simulink model "experiment_simulation"  (R2023b)
settings: Solver=VariableStepAuto  StartTime=0.0  StopTime=27  RelTol=1e-3
InitFcn:
  | parameters
model workspace (MAT data in the model file):
  trajectory_a = [-1.52409846931 0.800900294758 0.522291166812 0.881049446282 0.615681685123 0.846225707965 -1.91228070877 1.70613035573 -0.416782684687 1.94182780206 0.715113366686 0.630917086666 ... (70 elements, 7x10)]
  trajectory_b = [1.63785922603 1.06519745333 0.917286904974 -0.0990593700309 -1.33458996905 1.44935684592 -1.71486047215 -1.76858838765 1.00521664875 1.43938283234 1.2212819449 -1.40157163353 ... (70 elements, 7x10)]
values from neighbouring files (symbols this model uses):
  m = length(U)-1    [bspline_findspan.m]
  param_robot = load_mu(param_robot, mu)    [parameters.m]
undefined symbols (not defined in the file or in its folder): par, param_initial_condition, param_sensor, X, Y, Z
libraries: nesl_utility x308, sm_lib x269, simulink_extras x1
(part 3 of 4)

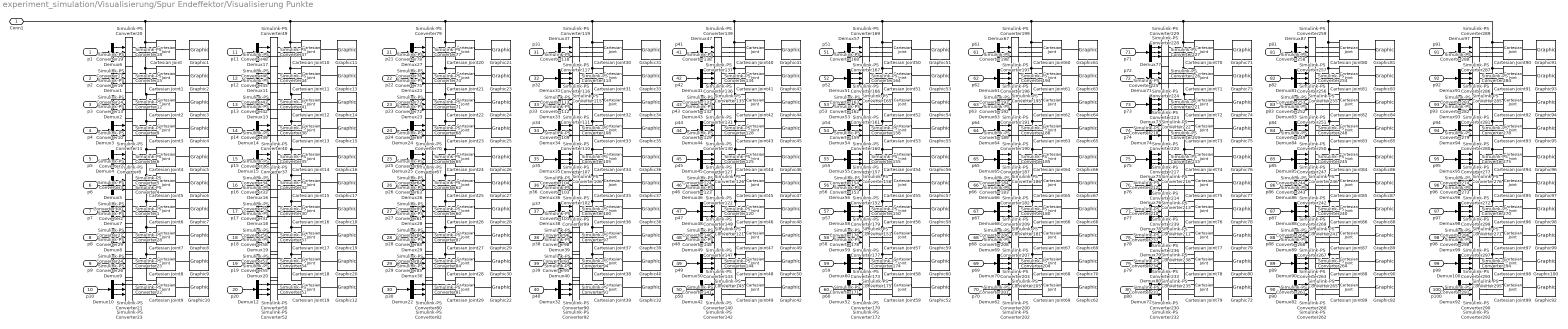
== system experiment_simulation/Visualisierung/Spur Endeffektor/Visualisierung Punkte ==
  p1 : Inport
  p2 : Inport  Port=2
  p3 : Inport  Port=3
  p4 : Inport  Port=4
  p5 : Inport  Port=5
  p6 : Inport  Port=6
  p7 : Inport  Port=7
  p8 : Inport  Port=8
  p9 : Inport  Port=9
  p10 : Inport  Port=10
  p11 : Inport  Port=11
  p12 : Inport  Port=12
  p13 : Inport  Port=13
  p14 : Inport  Port=14
  p15 : Inport  Port=15
  p16 : Inport  Port=16
  p17 : Inport  Port=17
  p18 : Inport  Port=18
  p19 : Inport  Port=19
  p20 : Inport  Port=20
  p21 : Inport  Port=21
  p22 : Inport  Port=22
  p23 : Inport  Port=23
  p24 : Inport  Port=24
  p25 : Inport  Port=25
  p26 : Inport  Port=26
  p27 : Inport  Port=27
  p28 : Inport  Port=28
  p29 : Inport  Port=29
  p30 : Inport  Port=30
  p31 : Inport  Port=31
  p32 : Inport  Port=32
  p33 : Inport  Port=33
  p34 : Inport  Port=34
  p35 : Inport  Port=35
  p36 : Inport  Port=36
  p37 : Inport  Port=37
  p38 : Inport  Port=38
  p39 : Inport  Port=39
  p40 : Inport  Port=40
  p41 : Inport  Port=41
  p42 : Inport  Port=42
  p43 : Inport  Port=43
  p44 : Inport  Port=44
  p45 : Inport  Port=45
  p46 : Inport  Port=46
  p47 : Inport  Port=47
  p48 : Inport  Port=48
  p49 : Inport  Port=49
  p50 : Inport  Port=50
  p51 : Inport  Port=51
  p52 : Inport  Port=52
  p53 : Inport  Port=53
  p54 : Inport  Port=54
  p55 : Inport  Port=55
  p56 : Inport  Port=56
  p57 : Inport  Port=57
  p58 : Inport  Port=58
  p59 : Inport  Port=59
  p60 : Inport  Port=60
  p61 : Inport  Port=61
  p62 : Inport  Port=62
  p63 : Inport  Port=63
  p64 : Inport  Port=64
  p65 : Inport  Port=65
  p66 : Inport  Port=66
  p67 : Inport  Port=67
  p68 : Inport  Port=68
  p69 : Inport  Port=69
  p70 : Inport  Port=70
  p71 : Inport  Port=71
  p72 : Inport  Port=72
  p73 : Inport  Port=73
  p74 : Inport  Port=74
  p75 : Inport  Port=75
  p76 : Inport  Port=76
  p77 : Inport  Port=77
  p78 : Inport  Port=78
  p79 : Inport  Port=79
  p80 : Inport  Port=80
  p81 : Inport  Port=81
  p82 : Inport  Port=82
  p83 : Inport  Port=83
  p84 : Inport  Port=84
  p85 : Inport  Port=85
  p86 : Inport  Port=86
  p87 : Inport  Port=87
  p88 : Inport  Port=88
  p89 : Inport  Port=89
  p90 : Inport  Port=90
  p91 : Inport  Port=91
  p92 : Inport  Port=92
  p93 : Inport  Port=93
  p94 : Inport  Port=94
  p95 : Inport  Port=95
  p96 : Inport  Port=96
  p97 : Inport  Port=97
  p98 : Inport  Port=98
  p99 : Inport  Port=99
  p100 : Inport  Port=100
  Cartesian Joint{,1..99} (100 alike) : sm_lib/Joints/Cartesian Joint  JointMode=Normal  SenseConstraintForce=off  SenseConstraintForceX=off  SenseConstraintForceY=off  SenseConstraintForceZ=off  SenseConstraintTorque=off  SenseConstraintTorqueX=off  SenseConstraintTorqueY=off  SenseConstraintTorqueZ=off  SenseTotalForce=off  SenseTotalForceX=off  SenseTotalForceY=off  SenseTotalForceZ=off  SenseTotalTorque=off  SenseTotalTorqueX=off  SenseTotalTorqueY=off  SenseTotalTorqueZ=off  CompositeWrenchDir=FollowerOnBase  CompositeWrenchFrame=BaseFrame  PxEquilibriumPosition=0  PxEquilibriumPositionUnits=m  PxSpringStiffness=0  PxSpringStiffnessUnits=N/m  PxDampingCoefficient=0  PxDampingCoefficientUnits=N/(m/s)  PxTorqueActuationMode=ComputedTorque  PxMotionActuationMode=InputMotion  PxSensePosition=off  PxSenseVelocity=off  PxSenseAcceleration=off  PxSenseTorqueForce=off  PxSenseLowerLimitTorqueForce=off  PxSenseUpperLimitTorqueForce=off  PxLowerLimitSpecify=off  PxLowerLimitBound=-1  PxLowerLimitBoundUnits=m  PxLowerLimitStiffness=1e6  PxLowerLimitStiffnessUnits=N/m  PxLowerLimitDamping=1e3  PxLowerLimitDampingUnits=N/(m/s)  PxLowerLimitTransitionRegionWidth=1e-4  PxLowerLimitTransitionRegionWidthUnits=m  PxUpperLimitSpecify=off  PxUpperLimitBound=1  PxUpperLimitBoundUnits=m  PxUpperLimitStiffness=1e6  PxUpperLimitStiffnessUnits=N/m  PxUpperLimitDamping=1e3  PxUpperLimitDampingUnits=N/(m/s)  PxUpperLimitTransitionRegionWidth=1e-4  PxUpperLimitTransitionRegionWidthUnits=m  PxPositionTargetSpecify=off  PxPositionTargetPriority=High  PxPositionTargetValue=0  PxPositionTargetValueUnits=m  PxVelocityTargetSpecify=off  PxVelocityTargetPriority=High  PxVelocityTargetValue=0  PxVelocityTargetValueUnits=m/s  PyEquilibriumPosition=0  PyEquilibriumPositionUnits=m  PySpringStiffness=0  PySpringStiffnessUnits=N/m  PyDampingCoefficient=0  PyDampingCoefficientUnits=N/(m/s)  PyTorqueActuationMode=ComputedTorque  PyMotionActuationMode=InputMotion  PySensePosition=off  PySenseVelocity=off  PySenseAcceleration=off  PySenseTorqueForce=off  PySenseLowerLimitTorqueForce=off  PySenseUpperLimitTorqueForce=off  PyLowerLimitSpecify=off  PyLowerLimitBound=-1  PyLowerLimitBoundUnits=m  PyLowerLimitStiffness=1e6  PyLowerLimitStiffnessUnits=N/m  PyLowerLimitDamping=1e3  PyLowerLimitDampingUnits=N/(m/s)  PyLowerLimitTransitionRegionWidth=1e-4  PyLowerLimitTransitionRegionWidthUnits=m  PyUpperLimitSpecify=off  PyUpperLimitBound=1  PyUpperLimitBoundUnits=m  PyUpperLimitStiffness=1e6  PyUpperLimitStiffnessUnits=N/m  PyUpperLimitDamping=1e3  PyUpperLimitDampingUnits=N/(m/s)  PyUpperLimitTransitionRegionWidth=1e-4  PyUpperLimitTransitionRegionWidthUnits=m  PyPositionTargetSpecify=off  PyPositionTargetPriority=High  PyPositionTargetValue=0  PyPositionTargetValueUnits=m  PyVelocityTargetSpecify=off  PyVelocityTargetPriority=High  PyVelocityTargetValue=0  PyVelocityTargetValueUnits=m/s  PzEquilibriumPosition=0  PzEquilibriumPositionUnits=m  PzSpringStiffness=0  PzSpringStiffnessUnits=N/m  PzDampingCoefficient=0  PzDampingCoefficientUnits=N/(m/s)  PzTorqueActuationMode=ComputedTorque  PzMotionActuationMode=InputMotion  PzSensePosition=off  PzSenseVelocity=off  PzSenseAcceleration=off  PzSenseTorqueForce=off  PzSenseLowerLimitTorqueForce=off  PzSenseUpperLimitTorqueForce=off  PzLowerLimitSpecify=off  PzLowerLimitBound=-1  PzLowerLimitBoundUnits=m  PzLowerLimitStiffness=1e6  PzLowerLimitStiffnessUnits=N/m  PzLowerLimitDamping=1e3  PzLowerLimitDampingUnits=N/(m/s)  PzLowerLimitTransitionRegionWidth=1e-4  PzLowerLimitTransitionRegionWidthUnits=m  PzUpperLimitSpecify=off  PzUpperLimitBound=1  PzUpperLimitBoundUnits=m  PzUpperLimitStiffness=1e6  PzUpperLimitStiffnessUnits=N/m  PzUpperLimitDamping=1e3  PzUpperLimitDampingUnits=N/(m/s)  PzUpperLimitTransitionRegionWidth=1e-4  PzUpperLimitTransitionRegionWidthUnits=m  PzPositionTargetSpecify=off  PzPositionTargetPriority=High  PzPositionTargetValue=0  PzPositionTargetValueUnits=m  PzVelocityTargetSpecify=off  PzVelocityTargetPriority=High  PzVelocityTargetValue=0  PzVelocityTargetValueUnits=m/s
  Demux{1..100} (100 alike) : Demux  Outputs=3
  Graphic{1..100} (100 alike) : sm_lib/Body Elements/Graphic  GraphicType=Marker  MarkerShape=Sphere  MarkerSize=par.vis_point.pix  GraphicVisPropType=SimpleVisualProperties  GraphicDiffuseColor=par.vis_point.col  GraphicSpecularColor=[0.5 0.5 0.5 1.0]  GraphicAmbientColor=[0.15 0.15 0.15 1.0]  GraphicEmissiveColor=[0.0 0.0 0.0 1.0]  GraphicShininess=75  GraphicOpacity=par.vis_point.opa
  Simulink-PS Converter{1..300} (300 alike) : nesl_utility/Simulink-PS Converter  PhysicalDomain=network_engine_domain  SubClassName=ps_input  LeftPortType=input  RightPortType=output  PseudoPeriodic=off  Frequencies=[]  NoiseDistribution=none  NoiseParameters=[]  Unit=1  AffineConversion=off  FilteringAndDerivatives=zero  SimscapeFilterOrder=2  InputFilterTimeConstant=0.001  UdotUserProvided=0
  Conn1 : PMIOPort  Side=Left
  wires:
  Demux6/2 -> Simulink-PS Converter18/1
  Demux6/3 -> Simulink-PS Converter19/1
  Demux6/1 -> Simulink-PS Converter20/1
  p1/1 -> Demux6/1
  Demux1/3 -> Simulink-PS Converter16/1
  Demux1/1 -> Simulink-PS Converter17/1
  Demux1/2 -> Simulink-PS Converter15/1
  p2/1 -> Demux1/1
  Demux2/3 -> Simulink-PS Converter13/1
  Demux2/1 -> Simulink-PS Converter14/1
  Demux2/2 -> Simulink-PS Converter12/1
  p3/1 -> Demux2/1
  Demux3/3 -> Simulink-PS Converter10/1
  Demux3/1 -> Simulink-PS Converter11/1
  Demux3/2 -> Simulink-PS Converter9/1
  p4/1 -> Demux3/1
  Demux4/3 -> Simulink-PS Converter7/1
  Demux4/1 -> Simulink-PS Converter8/1
  Demux4/2 -> Simulink-PS Converter6/1
  p5/1 -> Demux4/1
  Demux5/3 -> Simulink-PS Converter4/1
  Demux5/1 -> Simulink-PS Converter5/1
  Demux5/2 -> Simulink-PS Converter3/1
  p6/1 -> Demux5/1
  Demux7/3 -> Simulink-PS Converter2/1
  Demux7/1 -> Simulink-PS Converter300/1
  Demux7/2 -> Simulink-PS Converter1/1
  p7/1 -> Demux7/1
  Demux8/3 -> Simulink-PS Converter29/1
  Demux8/1 -> Simulink-PS Converter27/1
  Demux8/2 -> Simulink-PS Converter28/1
  p8/1 -> Demux8/1
  Demux9/3 -> Simulink-PS Converter26/1
  Demux9/1 -> Simulink-PS Converter24/1
  Demux9/2 -> Simulink-PS Converter25/1
  p9/1 -> Demux9/1
  Demux10/3 -> Simulink-PS Converter23/1
  Demux10/1 -> Simulink-PS Converter21/1
  Demux10/2 -> Simulink-PS Converter22/1
  p10/1 -> Demux10/1
  Demux16/2 -> Simulink-PS Converter32/1
  Demux16/1 -> Simulink-PS Converter34/1
  p16/1 -> Demux16/1
  p20/1 -> Demux12/1
  Demux12/2 -> Simulink-PS Converter51/1
  Demux12/1 -> Simulink-PS Converter50/1
  Demux12/3 -> Simulink-PS Converter52/1
  Demux17/1 -> Simulink-PS Converter49/1
  Demux17/3 -> Simulink-PS Converter48/1
  Demux17/2 -> Simulink-PS Converter47/1
  p11/1 -> Demux17/1
  Demux19/3 -> Simulink-PS Converter58/1
  p18/1 -> Demux19/1
  Demux11/2 -> Simulink-PS Converter44/1
  Demux11/1 -> Simulink-PS Converter46/1
  Demux19/2 -> Simulink-PS Converter57/1
  Demux11/3 -> Simulink-PS Converter45/1
  Demux19/1 -> Simulink-PS Converter56/1
  Demux15/1 -> Simulink-PS Converter37/1
  p12/1 -> Demux11/1
  p15/1 -> Demux15/1
  p17/1 -> Demux18/1
  Demux18/2 -> Simulink-PS Converter30/1
  Demux18/3 -> Simulink-PS Converter31/1
  Demux18/1 -> Simulink-PS Converter59/1
  Demux13/2 -> Simulink-PS Converter41/1
  Demux15/2 -> Simulink-PS Converter35/1
  Demux14/3 -> Simulink-PS Converter39/1
  Demux13/1 -> Simulink-PS Converter43/1
  Demux13/3 -> Simulink-PS Converter42/1
  Demux14/2 -> Simulink-PS Converter38/1
  Demux16/3 -> Simulink-PS Converter33/1
  p13/1 -> Demux13/1
  p19/1 -> Demux20/1
  Demux20/3 -> Simulink-PS Converter55/1
  p14/1 -> Demux14/1
  Demux20/1 -> Simulink-PS Converter53/1
  Demux14/1 -> Simulink-PS Converter40/1
  Demux20/2 -> Simulink-PS Converter54/1
  Demux15/3 -> Simulink-PS Converter36/1
  Demux26/2 -> Simulink-PS Converter62/1
  Demux26/1 -> Simulink-PS Converter64/1
  p26/1 -> Demux26/1
  p30/1 -> Demux22/1
  Demux22/2 -> Simulink-PS Converter81/1
  Demux22/1 -> Simulink-PS Converter80/1
  Demux22/3 -> Simulink-PS Converter82/1
  Demux27/1 -> Simulink-PS Converter79/1
  Demux27/3 -> Simulink-PS Converter78/1
  Demux27/2 -> Simulink-PS Converter77/1
  p21/1 -> Demux27/1
  Demux29/3 -> Simulink-PS Converter88/1
  p28/1 -> Demux29/1
  Demux21/2 -> Simulink-PS Converter74/1
  Demux21/1 -> Simulink-PS Converter76/1
  Demux29/2 -> Simulink-PS Converter87/1
  Demux21/3 -> Simulink-PS Converter75/1
  Demux29/1 -> Simulink-PS Converter86/1
  Demux25/1 -> Simulink-PS Converter67/1
  p22/1 -> Demux21/1
  p25/1 -> Demux25/1
  p27/1 -> Demux28/1
  Demux28/2 -> Simulink-PS Converter60/1
  Demux28/3 -> Simulink-PS Converter61/1
  Demux28/1 -> Simulink-PS Converter89/1
  Demux23/2 -> Simulink-PS Converter71/1
  Demux25/2 -> Simulink-PS Converter65/1
  Demux24/3 -> Simulink-PS Converter69/1
  Demux23/1 -> Simulink-PS Converter73/1
  Demux23/3 -> Simulink-PS Converter72/1
  Demux24/2 -> Simulink-PS Converter68/1
  Demux26/3 -> Simulink-PS Converter63/1
  p23/1 -> Demux23/1
  p29/1 -> Demux30/1
  Demux30/3 -> Simulink-PS Converter85/1
  p24/1 -> Demux24/1
  Demux30/1 -> Simulink-PS Converter83/1
  Demux24/1 -> Simulink-PS Converter70/1
  Demux30/2 -> Simulink-PS Converter84/1
  Demux25/3 -> Simulink-PS Converter66/1
  Demux36/2 -> Simulink-PS Converter102/1
  Demux36/1 -> Simulink-PS Converter104/1
  p36/1 -> Demux36/1
  p40/1 -> Demux32/1
  Demux32/2 -> Simulink-PS Converter91/1
  Demux32/1 -> Simulink-PS Converter90/1
  Demux32/3 -> Simulink-PS Converter92/1
  Demux37/1 -> Simulink-PS Converter119/1
  Demux37/3 -> Simulink-PS Converter118/1
  Demux37/2 -> Simulink-PS Converter117/1
  p31/1 -> Demux37/1
  Demux39/3 -> Simulink-PS Converter98/1
  p38/1 -> Demux39/1
  Demux31/2 -> Simulink-PS Converter114/1
  Demux31/1 -> Simulink-PS Converter116/1
  Demux39/2 -> Simulink-PS Converter97/1
  Demux31/3 -> Simulink-PS Converter115/1
  Demux39/1 -> Simulink-PS Converter96/1
  Demux35/1 -> Simulink-PS Converter107/1
  p32/1 -> Demux31/1
  p35/1 -> Demux35/1
  p37/1 -> Demux38/1
  Demux38/2 -> Simulink-PS Converter100/1
  Demux38/3 -> Simulink-PS Converter101/1
  Demux38/1 -> Simulink-PS Converter99/1
  Demux33/2 -> Simulink-PS Converter111/1
  Demux35/2 -> Simulink-PS Converter105/1
  Demux34/3 -> Simulink-PS Converter109/1
  Demux33/1 -> Simulink-PS Converter113/1
  Demux33/3 -> Simulink-PS Converter112/1
  Demux34/2 -> Simulink-PS Converter108/1
  Demux36/3 -> Simulink-PS Converter103/1
  p33/1 -> Demux33/1
  p39/1 -> Demux40/1
  Demux40/3 -> Simulink-PS Converter95/1
  p34/1 -> Demux34/1
  Demux40/1 -> Simulink-PS Converter93/1
  Demux34/1 -> Simulink-PS Converter110/1
  Demux40/2 -> Simulink-PS Converter94/1
  Demux35/3 -> Simulink-PS Converter106/1
  Demux46/2 -> Simulink-PS Converter122/1
  Demux46/1 -> Simulink-PS Converter124/1
  p46/1 -> Demux46/1
  p50/1 -> Demux42/1
  Demux42/2 -> Simulink-PS Converter141/1
  Demux42/1 -> Simulink-PS Converter140/1
  Demux42/3 -> Simulink-PS Converter142/1
  Demux47/1 -> Simulink-PS Converter139/1
  Demux47/3 -> Simulink-PS Converter138/1
  Demux47/2 -> Simulink-PS Converter137/1
  p41/1 -> Demux47/1
  Demux49/3 -> Simulink-PS Converter148/1
  p48/1 -> Demux49/1
  Demux41/2 -> Simulink-PS Converter134/1
  Demux41/1 -> Simulink-PS Converter136/1
  Demux49/2 -> Simulink-PS Converter147/1
  Demux41/3 -> Simulink-PS Converter135/1
  Demux49/1 -> Simulink-PS Converter146/1
  Demux45/1 -> Simulink-PS Converter127/1
  p42/1 -> Demux41/1
  p45/1 -> Demux45/1
  p47/1 -> Demux48/1
  Demux48/2 -> Simulink-PS Converter120/1
  Demux48/3 -> Simulink-PS Converter121/1
  Demux48/1 -> Simulink-PS Converter149/1
  Demux43/2 -> Simulink-PS Converter131/1
  Demux45/2 -> Simulink-PS Converter125/1
  Demux44/3 -> Simulink-PS Converter129/1
  Demux43/1 -> Simulink-PS Converter133/1
  Demux43/3 -> Simulink-PS Converter132/1
  Demux44/2 -> Simulink-PS Converter128/1
  Demux46/3 -> Simulink-PS Converter123/1
  p43/1 -> Demux43/1
  p49/1 -> Demux50/1
  Demux50/3 -> Simulink-PS Converter145/1
  p44/1 -> Demux44/1
  Demux50/1 -> Simulink-PS Converter143/1
  Demux44/1 -> Simulink-PS Converter130/1
  Demux50/2 -> Simulink-PS Converter144/1
  Demux45/3 -> Simulink-PS Converter126/1
  Demux56/2 -> Simulink-PS Converter152/1
  Demux56/1 -> Simulink-PS Converter154/1
  p56/1 -> Demux56/1
  p60/1 -> Demux52/1
  Demux52/2 -> Simulink-PS Converter171/1
  Demux52/1 -> Simulink-PS Converter170/1
  Demux52/3 -> Simulink-PS Converter172/1
  Demux57/1 -> Simulink-PS Converter169/1
  Demux57/3 -> Simulink-PS Converter168/1
  Demux57/2 -> Simulink-PS Converter167/1
  p51/1 -> Demux57/1
  Demux59/3 -> Simulink-PS Converter178/1
  p58/1 -> Demux59/1
  Demux51/2 -> Simulink-PS Converter164/1
  Demux51/1 -> Simulink-PS Converter166/1
  Demux59/2 -> Simulink-PS Converter177/1
  Demux51/3 -> Simulink-PS Converter165/1
  Demux59/1 -> Simulink-PS Converter176/1
  Demux55/1 -> Simulink-PS Converter157/1
  p52/1 -> Demux51/1
  p55/1 -> Demux55/1
  p57/1 -> Demux58/1
  Demux58/2 -> Simulink-PS Converter150/1
  Demux58/3 -> Simulink-PS Converter151/1
  Demux58/1 -> Simulink-PS Converter179/1
  Demux53/2 -> Simulink-PS Converter161/1
  Demux55/2 -> Simulink-PS Converter155/1
  Demux54/3 -> Simulink-PS Converter159/1
  Demux53/1 -> Simulink-PS Converter163/1
  Demux53/3 -> Simulink-PS Converter162/1
  Demux54/2 -> Simulink-PS Converter158/1
  Demux56/3 -> Simulink-PS Converter153/1
  p53/1 -> Demux53/1
  p59/1 -> Demux60/1
  Demux60/3 -> Simulink-PS Converter175/1
  p54/1 -> Demux54/1
  Demux60/1 -> Simulink-PS Converter173/1
  Demux54/1 -> Simulink-PS Converter160/1
  Demux60/2 -> Simulink-PS Converter174/1
  Demux55/3 -> Simulink-PS Converter156/1
  Demux66/2 -> Simulink-PS Converter182/1
  Demux66/1 -> Simulink-PS Converter184/1
  p66/1 -> Demux66/1
  p70/1 -> Demux62/1
  Demux62/2 -> Simulink-PS Converter201/1
  Demux62/1 -> Simulink-PS Converter200/1
  Demux62/3 -> Simulink-PS Converter202/1
  Demux67/1 -> Simulink-PS Converter199/1
  Demux67/3 -> Simulink-PS Converter198/1
  Demux67/2 -> Simulink-PS Converter197/1
  p61/1 -> Demux67/1
  Demux69/3 -> Simulink-PS Converter208/1
  p68/1 -> Demux69/1
  Demux61/2 -> Simulink-PS Converter194/1
  Demux61/1 -> Simulink-PS Converter196/1
  Demux69/2 -> Simulink-PS Converter207/1
  Demux61/3 -> Simulink-PS Converter195/1
  Demux69/1 -> Simulink-PS Converter206/1
  Demux65/1 -> Simulink-PS Converter187/1
  p62/1 -> Demux61/1
  p65/1 -> Demux65/1
  p67/1 -> Demux68/1
  Demux68/2 -> Simulink-PS Converter180/1
  Demux68/3 -> Simulink-PS Converter181/1
  Demux68/1 -> Simulink-PS Converter209/1
  Demux63/2 -> Simulink-PS Converter191/1
  Demux65/2 -> Simulink-PS Converter185/1
  Demux64/3 -> Simulink-PS Converter189/1
  Demux63/1 -> Simulink-PS Converter193/1
  Demux63/3 -> Simulink-PS Converter192/1
  Demux64/2 -> Simulink-PS Converter188/1
  Demux66/3 -> Simulink-PS Converter183/1
  p63/1 -> Demux63/1
  p69/1 -> Demux70/1
  Demux70/3 -> Simulink-PS Converter205/1
  p64/1 -> Demux64/1
  Demux70/1 -> Simulink-PS Converter203/1
  Demux64/1 -> Simulink-PS Converter190/1
  Demux70/2 -> Simulink-PS Converter204/1
  Demux65/3 -> Simulink-PS Converter186/1
  Demux76/2 -> Simulink-PS Converter212/1
  Demux76/1 -> Simulink-PS Converter214/1
  p76/1 -> Demux76/1
  p80/1 -> Demux72/1
  Demux72/2 -> Simulink-PS Converter231/1
  Demux72/1 -> Simulink-PS Converter230/1
  Demux72/3 -> Simulink-PS Converter232/1
  Demux77/1 -> Simulink-PS Converter229/1
  Demux77/3 -> Simulink-PS Converter228/1
  Demux77/2 -> Simulink-PS Converter227/1
  p71/1 -> Demux77/1
  Demux79/3 -> Simulink-PS Converter238/1
  p78/1 -> Demux79/1
  Demux71/2 -> Simulink-PS Converter224/1
  Demux71/1 -> Simulink-PS Converter226/1
  Demux79/2 -> Simulink-PS Converter237/1
  Demux71/3 -> Simulink-PS Converter225/1
  Demux79/1 -> Simulink-PS Converter236/1
  Demux75/1 -> Simulink-PS Converter217/1
  p72/1 -> Demux71/1
  p75/1 -> Demux75/1
  p77/1 -> Demux78/1
  Demux78/2 -> Simulink-PS Converter210/1
  Demux78/3 -> Simulink-PS Converter211/1
  Demux78/1 -> Simulink-PS Converter239/1
  Demux73/2 -> Simulink-PS Converter221/1
  Demux75/2 -> Simulink-PS Converter215/1
  Demux74/3 -> Simulink-PS Converter219/1
  Demux73/1 -> Simulink-PS Converter223/1
  Demux73/3 -> Simulink-PS Converter222/1
  Demux74/2 -> Simulink-PS Converter218/1
  Demux76/3 -> Simulink-PS Converter213/1
  p73/1 -> Demux73/1
  p79/1 -> Demux80/1
  Demux80/3 -> Simulink-PS Converter235/1
  p74/1 -> Demux74/1
  Demux80/1 -> Simulink-PS Converter233/1
  Demux74/1 -> Simulink-PS Converter220/1
  Demux80/2 -> Simulink-PS Converter234/1
  Demux75/3 -> Simulink-PS Converter216/1
  Demux86/2 -> Simulink-PS Converter242/1
  Demux86/1 -> Simulink-PS Converter244/1
  p86/1 -> Demux86/1
  p90/1 -> Demux82/1
  Demux82/2 -> Simulink-PS Converter261/1
  Demux82/1 -> Simulink-PS Converter260/1
  Demux82/3 -> Simulink-PS Converter262/1
  Demux87/1 -> Simulink-PS Converter259/1
  Demux87/3 -> Simulink-PS Converter258/1
  Demux87/2 -> Simulink-PS Converter257/1
  p81/1 -> Demux87/1
  Demux89/3 -> Simulink-PS Converter268/1
  p88/1 -> Demux89/1
  Demux81/2 -> Simulink-PS Converter254/1
  Demux81/1 -> Simulink-PS Converter256/1
  Demux89/2 -> Simulink-PS Converter267/1
  Demux81/3 -> Simulink-PS Converter255/1
  Demux89/1 -> Simulink-PS Converter266/1
  Demux85/1 -> Simulink-PS Converter247/1
  p82/1 -> Demux81/1
  p85/1 -> Demux85/1
  p87/1 -> Demux88/1
  Demux88/2 -> Simulink-PS Converter240/1
  Demux88/3 -> Simulink-PS Converter241/1
  Demux88/1 -> Simulink-PS Converter269/1
  Demux83/2 -> Simulink-PS Converter251/1
  Demux85/2 -> Simulink-PS Converter245/1
  Demux84/3 -> Simulink-PS Converter249/1
  Demux83/1 -> Simulink-PS Converter253/1
  Demux83/3 -> Simulink-PS Converter252/1
  Demux84/2 -> Simulink-PS Converter248/1
  Demux86/3 -> Simulink-PS Converter243/1
  p83/1 -> Demux83/1
  p89/1 -> Demux90/1
  Demux90/3 -> Simulink-PS Converter265/1
  p84/1 -> Demux84/1
  Demux90/1 -> Simulink-PS Converter263/1
  Demux84/1 -> Simulink-PS Converter250/1
  Demux90/2 -> Simulink-PS Converter264/1
  Demux85/3 -> Simulink-PS Converter246/1
  Demux96/2 -> Simulink-PS Converter272/1
  Demux96/1 -> Simulink-PS Converter274/1
  p96/1 -> Demux96/1
  p100/1 -> Demux92/1
  Demux92/2 -> Simulink-PS Converter291/1
  Demux92/1 -> Simulink-PS Converter290/1
  Demux92/3 -> Simulink-PS Converter292/1
  Demux97/1 -> Simulink-PS Converter289/1
  Demux97/3 -> Simulink-PS Converter288/1
  Demux97/2 -> Simulink-PS Converter287/1
  p91/1 -> Demux97/1
  Demux99/3 -> Simulink-PS Converter298/1
  p98/1 -> Demux99/1
  Demux91/2 -> Simulink-PS Converter284/1
  Demux91/1 -> Simulink-PS Converter286/1
  Demux99/2 -> Simulink-PS Converter297/1
  Demux91/3 -> Simulink-PS Converter285/1
  Demux99/1 -> Simulink-PS Converter296/1
  Demux95/1 -> Simulink-PS Converter277/1
  p92/1 -> Demux91/1
  p95/1 -> Demux95/1
  p97/1 -> Demux98/1
  Demux98/2 -> Simulink-PS Converter270/1
  Demux98/3 -> Simulink-PS Converter271/1
  Demux98/1 -> Simulink-PS Converter299/1
  Demux93/2 -> Simulink-PS Converter281/1
  Demux95/2 -> Simulink-PS Converter275/1
  Demux94/3 -> Simulink-PS Converter279/1
  Demux93/1 -> Simulink-PS Converter283/1
  Demux93/3 -> Simulink-PS Converter282/1
  Demux94/2 -> Simulink-PS Converter278/1
  Demux96/3 -> Simulink-PS Converter273/1
  p93/1 -> Demux93/1
  p99/1 -> Demux100/1
  Demux100/3 -> Simulink-PS Converter295/1
  p94/1 -> Demux94/1
  Demux100/1 -> Simulink-PS Converter293/1
  Demux94/1 -> Simulink-PS Converter280/1
  Demux100/2 -> Simulink-PS Converter294/1
  Demux95/3 -> Simulink-PS Converter276/1
  connections:
  Simulink-PS Converter18/RConn1 -- Cartesian Joint/LConn3
  Simulink-PS Converter19/RConn1 -- Cartesian Joint/LConn4
  Cartesian Joint/RConn1 -- Graphic1/RConn1
  Simulink-PS Converter20/RConn1 -- Cartesian Joint/LConn2
  Cartesian Joint92/LConn1 -- Cartesian Joint98/LConn1 -- Cartesian Joint99/LConn1 -- Cartesian Joint97/LConn1 -- Cartesian Joint96/LConn1 -- Cartesian Joint95/LConn1 -- Cartesian Joint94/LConn1 -- Cartesian Joint93/LConn1 -- Conn1/RConn1 -- Cartesian Joint8/LConn1 -- Cartesian Joint9/LConn1 -- Cartesian Joint7/LConn1 -- Cartesian Joint6/LConn1 -- Cartesian Joint5/LConn1 -- Cartesian Joint4/LConn1 -- Cartesian Joint3/LConn1 -- Cartesian Joint2/LConn1 -- Cartesian Joint1/LConn1 -- Cartesian Joint/LConn1 -- Cartesian Joint10/LConn1 -- Cartesian Joint11/LConn1 -- Cartesian Joint18/LConn1 -- Cartesian Joint19/LConn1 -- Cartesian Joint17/LConn1 -- Cartesian Joint16/LConn1 -- Cartesian Joint15/LConn1 -- Cartesian Joint14/LConn1 -- Cartesian Joint13/LConn1 -- Cartesian Joint12/LConn1 -- Cartesian Joint20/LConn1 -- Cartesian Joint21/LConn1 -- Cartesian Joint28/LConn1 -- Cartesian Joint29/LConn1 -- Cartesian Joint27/LConn1 -- Cartesian Joint26/LConn1 -- Cartesian Joint25/LConn1 -- Cartesian Joint24/LConn1 -- Cartesian Joint23/LConn1 -- Cartesian Joint22/LConn1 -- Cartesian Joint30/LConn1 -- Cartesian Joint31/LConn1 -- Cartesian Joint38/LConn1 -- Cartesian Joint39/LConn1 -- Cartesian Joint37/LConn1 -- Cartesian Joint36/LConn1 -- Cartesian Joint35/LConn1 -- Cartesian Joint34/LConn1 -- Cartesian Joint33/LConn1 -- Cartesian Joint32/LConn1 -- Cartesian Joint40/LConn1 -- Cartesian Joint41/LConn1 -- Cartesian Joint48/LConn1 -- Cartesian Joint49/LConn1 -- Cartesian Joint47/LConn1 -- Cartesian Joint46/LConn1 -- Cartesian Joint45/LConn1 -- Cartesian Joint44/LConn1 -- Cartesian Joint43/LConn1 -- Cartesian Joint42/LConn1 -- Cartesian Joint50/LConn1 -- Cartesian Joint51/LConn1 -- Cartesian Joint58/LConn1 -- Cartesian Joint59/LConn1 -- Cartesian Joint57/LConn1 -- Cartesian Joint56/LConn1 -- Cartesian Joint55/LConn1 -- Cartesian Joint54/LConn1 -- Cartesian Joint53/LConn1 -- Cartesian Joint52/LConn1 -- Cartesian Joint60/LConn1 -- Cartesian Joint61/LConn1 -- Cartesian Joint68/LConn1 -- Cartesian Joint69/LConn1 -- Cartesian Joint67/LConn1 -- Cartesian Joint66/LConn1 -- Cartesian Joint65/LConn1 -- Cartesian Joint64/LConn1 -- Cartesian Joint63/LConn1 -- Cartesian Joint62/LConn1 -- Cartesian Joint70/LConn1 -- Cartesian Joint71/LConn1 -- Cartesian Joint78/LConn1 -- Cartesian Joint79/LConn1 -- Cartesian Joint77/LConn1 -- Cartesian Joint76/LConn1 -- Cartesian Joint75/LConn1 -- Cartesian Joint74/LConn1 -- Cartesian Joint73/LConn1 -- Cartesian Joint72/LConn1 -- Cartesian Joint80/LConn1 -- Cartesian Joint81/LConn1 -- Cartesian Joint88/LConn1 -- Cartesian Joint89/LConn1 -- Cartesian Joint87/LConn1 -- Cartesian Joint86/LConn1 -- Cartesian Joint85/LConn1 -- Cartesian Joint84/LConn1 -- Cartesian Joint83/LConn1 -- Cartesian Joint82/LConn1 -- Cartesian Joint90/LConn1 -- Cartesian Joint91/LConn1
  Graphic2/RConn1 -- Cartesian Joint1/RConn1
  Graphic3/RConn1 -- Cartesian Joint2/RConn1
  Graphic4/RConn1 -- Cartesian Joint3/RConn1
  Graphic6/RConn1 -- Cartesian Joint5/RConn1
  Graphic7/RConn1 -- Cartesian Joint6/RConn1
  Graphic8/RConn1 -- Cartesian Joint7/RConn1
  Graphic5/RConn1 -- Cartesian Joint4/RConn1
  Graphic9/RConn1 -- Cartesian Joint8/RConn1
  Graphic10/RConn1 -- Cartesian Joint9/RConn1
  Simulink-PS Converter17/RConn1 -- Cartesian Joint1/LConn2
  Simulink-PS Converter16/RConn1 -- Cartesian Joint1/LConn4
  Simulink-PS Converter15/RConn1 -- Cartesian Joint1/LConn3
  Simulink-PS Converter14/RConn1 -- Cartesian Joint2/LConn2
  Simulink-PS Converter13/RConn1 -- Cartesian Joint2/LConn4
  Simulink-PS Converter12/RConn1 -- Cartesian Joint2/LConn3
  Simulink-PS Converter11/RConn1 -- Cartesian Joint3/LConn2
  Simulink-PS Converter10/RConn1 -- Cartesian Joint3/LConn4
  Simulink-PS Converter9/RConn1 -- Cartesian Joint3/LConn3
  Simulink-PS Converter8/RConn1 -- Cartesian Joint4/LConn2
  Simulink-PS Converter7/RConn1 -- Cartesian Joint4/LConn4
  Simulink-PS Converter6/RConn1 -- Cartesian Joint4/LConn3
  Simulink-PS Converter5/RConn1 -- Cartesian Joint5/LConn2
  Simulink-PS Converter4/RConn1 -- Cartesian Joint5/LConn4
  Simulink-PS Converter3/RConn1 -- Cartesian Joint5/LConn3
  Simulink-PS Converter300/RConn1 -- Cartesian Joint6/LConn2
  Simulink-PS Converter2/RConn1 -- Cartesian Joint6/LConn4
  Simulink-PS Converter1/RConn1 -- Cartesian Joint6/LConn3
  Simulink-PS Converter27/RConn1 -- Cartesian Joint7/LConn2
  Simulink-PS Converter29/RConn1 -- Cartesian Joint7/LConn4
  Simulink-PS Converter28/RConn1 -- Cartesian Joint7/LConn3
  Simulink-PS Converter24/RConn1 -- Cartesian Joint8/LConn2
  Simulink-PS Converter26/RConn1 -- Cartesian Joint8/LConn4
  Simulink-PS Converter25/RConn1 -- Cartesian Joint8/LConn3
  Simulink-PS Converter21/RConn1 -- Cartesian Joint9/LConn2
  Simulink-PS Converter23/RConn1 -- Cartesian Joint9/LConn4
  Simulink-PS Converter22/RConn1 -- Cartesian Joint9/LConn3
  Simulink-PS Converter53/RConn1 -- Cartesian Joint18/LConn2
  Simulink-PS Converter36/RConn1 -- Cartesian Joint14/LConn4
  Simulink-PS Converter41/RConn1 -- Cartesian Joint12/LConn3
  Simulink-PS Converter43/RConn1 -- Cartesian Joint12/LConn2
  Simulink-PS Converter52/RConn1 -- Cartesian Joint19/LConn4
  Simulink-PS Converter42/RConn1 -- Cartesian Joint12/LConn4
  Simulink-PS Converter50/RConn1 -- Cartesian Joint19/LConn2
  Simulink-PS Converter51/RConn1 -- Cartesian Joint19/LConn3
  Simulink-PS Converter37/RConn1 -- Cartesian Joint14/LConn2
  Simulink-PS Converter55/RConn1 -- Cartesian Joint18/LConn4
  Simulink-PS Converter32/RConn1 -- Cartesian Joint15/LConn3
  Graphic14/RConn1 -- Cartesian Joint12/RConn1
  Graphic12/RConn1 -- Cartesian Joint19/RConn1
  Simulink-PS Converter38/RConn1 -- Cartesian Joint13/LConn3
  Graphic15/RConn1 -- Cartesian Joint13/RConn1
  Simulink-PS Converter49/RConn1 -- Cartesian Joint10/LConn2
  Simulink-PS Converter56/RConn1 -- Cartesian Joint17/LConn2
  Simulink-PS Converter47/RConn1 -- Cartesian Joint10/LConn3
  Simulink-PS Converter33/RConn1 -- Cartesian Joint15/LConn4
  Graphic11/RConn1 -- Cartesian Joint10/RConn1
  Simulink-PS Converter34/RConn1 -- Cartesian Joint15/LConn2
  Simulink-PS Converter44/RConn1 -- Cartesian Joint11/LConn3
  Simulink-PS Converter31/RConn1 -- Cartesian Joint16/LConn4
  Simulink-PS Converter30/RConn1 -- Cartesian Joint16/LConn3
  Graphic18/RConn1 -- Cartesian Joint16/RConn1
  Graphic20/RConn1 -- Cartesian Joint18/RConn1
  Simulink-PS Converter39/RConn1 -- Cartesian Joint13/LConn4
  Simulink-PS Converter46/RConn1 -- Cartesian Joint11/LConn2
  Graphic17/RConn1 -- Cartesian Joint15/RConn1
  Simulink-PS Converter48/RConn1 -- Cartesian Joint10/LConn4
  Graphic16/RConn1 -- Cartesian Joint14/RConn1
  Graphic13/RConn1 -- Cartesian Joint11/RConn1
  Simulink-PS Converter35/RConn1 -- Cartesian Joint14/LConn3
  Simulink-PS Converter45/RConn1 -- Cartesian Joint11/LConn4
  Simulink-PS Converter59/RConn1 -- Cartesian Joint16/LConn2
  Simulink-PS Converter40/RConn1 -- Cartesian Joint13/LConn2
  Simulink-PS Converter58/RConn1 -- Cartesian Joint17/LConn4
  Graphic19/RConn1 -- Cartesian Joint17/RConn1
  Simulink-PS Converter57/RConn1 -- Cartesian Joint17/LConn3
  Simulink-PS Converter54/RConn1 -- Cartesian Joint18/LConn3
  Simulink-PS Converter83/RConn1 -- Cartesian Joint28/LConn2
  Simulink-PS Converter66/RConn1 -- Cartesian Joint24/LConn4
  Simulink-PS Converter71/RConn1 -- Cartesian Joint22/LConn3
  Simulink-PS Converter73/RConn1 -- Cartesian Joint22/LConn2
  Simulink-PS Converter82/RConn1 -- Cartesian Joint29/LConn4
  Simulink-PS Converter72/RConn1 -- Cartesian Joint22/LConn4
  Simulink-PS Converter80/RConn1 -- Cartesian Joint29/LConn2
  Simulink-PS Converter81/RConn1 -- Cartesian Joint29/LConn3
  Simulink-PS Converter67/RConn1 -- Cartesian Joint24/LConn2
  Simulink-PS Converter85/RConn1 -- Cartesian Joint28/LConn4
  Simulink-PS Converter62/RConn1 -- Cartesian Joint25/LConn3
  Graphic24/RConn1 -- Cartesian Joint22/RConn1
  Graphic22/RConn1 -- Cartesian Joint29/RConn1
  Simulink-PS Converter68/RConn1 -- Cartesian Joint23/LConn3
  Graphic25/RConn1 -- Cartesian Joint23/RConn1
  Simulink-PS Converter79/RConn1 -- Cartesian Joint20/LConn2
  Simulink-PS Converter86/RConn1 -- Cartesian Joint27/LConn2
  Simulink-PS Converter77/RConn1 -- Cartesian Joint20/LConn3
  Simulink-PS Converter63/RConn1 -- Cartesian Joint25/LConn4
  Graphic21/RConn1 -- Cartesian Joint20/RConn1
  Simulink-PS Converter64/RConn1 -- Cartesian Joint25/LConn2
  Simulink-PS Converter74/RConn1 -- Cartesian Joint21/LConn3
  Simulink-PS Converter61/RConn1 -- Cartesian Joint26/LConn4
  Simulink-PS Converter60/RConn1 -- Cartesian Joint26/LConn3
  Graphic28/RConn1 -- Cartesian Joint26/RConn1
  Graphic30/RConn1 -- Cartesian Joint28/RConn1
  Simulink-PS Converter69/RConn1 -- Cartesian Joint23/LConn4
  Simulink-PS Converter76/RConn1 -- Cartesian Joint21/LConn2
  Graphic27/RConn1 -- Cartesian Joint25/RConn1
  Simulink-PS Converter78/RConn1 -- Cartesian Joint20/LConn4
  Graphic26/RConn1 -- Cartesian Joint24/RConn1
  Graphic23/RConn1 -- Cartesian Joint21/RConn1
  Simulink-PS Converter65/RConn1 -- Cartesian Joint24/LConn3
  Simulink-PS Converter75/RConn1 -- Cartesian Joint21/LConn4
  Simulink-PS Converter89/RConn1 -- Cartesian Joint26/LConn2
  Simulink-PS Converter70/RConn1 -- Cartesian Joint23/LConn2
  Simulink-PS Converter88/RConn1 -- Cartesian Joint27/LConn4
  Graphic29/RConn1 -- Cartesian Joint27/RConn1
  Simulink-PS Converter87/RConn1 -- Cartesian Joint27/LConn3
  Simulink-PS Converter84/RConn1 -- Cartesian Joint28/LConn3
  Simulink-PS Converter93/RConn1 -- Cartesian Joint38/LConn2
  Simulink-PS Converter106/RConn1 -- Cartesian Joint34/LConn4
  Simulink-PS Converter111/RConn1 -- Cartesian Joint32/LConn3
  Simulink-PS Converter113/RConn1 -- Cartesian Joint32/LConn2
  Simulink-PS Converter92/RConn1 -- Cartesian Joint39/LConn4
  Simulink-PS Converter112/RConn1 -- Cartesian Joint32/LConn4
  Simulink-PS Converter90/RConn1 -- Cartesian Joint39/LConn2
  Simulink-PS Converter91/RConn1 -- Cartesian Joint39/LConn3
  Simulink-PS Converter107/RConn1 -- Cartesian Joint34/LConn2
  Simulink-PS Converter95/RConn1 -- Cartesian Joint38/LConn4
  Simulink-PS Converter102/RConn1 -- Cartesian Joint35/LConn3
  Graphic34/RConn1 -- Cartesian Joint32/RConn1
  Graphic32/RConn1 -- Cartesian Joint39/RConn1
  Simulink-PS Converter108/RConn1 -- Cartesian Joint33/LConn3
  Graphic35/RConn1 -- Cartesian Joint33/RConn1
  Simulink-PS Converter119/RConn1 -- Cartesian Joint30/LConn2
  Simulink-PS Converter96/RConn1 -- Cartesian Joint37/LConn2
  Simulink-PS Converter117/RConn1 -- Cartesian Joint30/LConn3
  Simulink-PS Converter103/RConn1 -- Cartesian Joint35/LConn4
  Graphic31/RConn1 -- Cartesian Joint30/RConn1
  Simulink-PS Converter104/RConn1 -- Cartesian Joint35/LConn2
  Simulink-PS Converter114/RConn1 -- Cartesian Joint31/LConn3
  Simulink-PS Converter101/RConn1 -- Cartesian Joint36/LConn4
  Simulink-PS Converter100/RConn1 -- Cartesian Joint36/LConn3
  Graphic38/RConn1 -- Cartesian Joint36/RConn1
  Graphic40/RConn1 -- Cartesian Joint38/RConn1
  Simulink-PS Converter109/RConn1 -- Cartesian Joint33/LConn4
  Simulink-PS Converter116/RConn1 -- Cartesian Joint31/LConn2
  Graphic37/RConn1 -- Cartesian Joint35/RConn1
  Simulink-PS Converter118/RConn1 -- Cartesian Joint30/LConn4
  Graphic36/RConn1 -- Cartesian Joint34/RConn1
  Graphic33/RConn1 -- Cartesian Joint31/RConn1
  Simulink-PS Converter105/RConn1 -- Cartesian Joint34/LConn3
  Simulink-PS Converter115/RConn1 -- Cartesian Joint31/LConn4
  Simulink-PS Converter99/RConn1 -- Cartesian Joint36/LConn2
  Simulink-PS Converter110/RConn1 -- Cartesian Joint33/LConn2
  Simulink-PS Converter98/RConn1 -- Cartesian Joint37/LConn4
  Graphic39/RConn1 -- Cartesian Joint37/RConn1
  Simulink-PS Converter97/RConn1 -- Cartesian Joint37/LConn3
  Simulink-PS Converter94/RConn1 -- Cartesian Joint38/LConn3
  Simulink-PS Converter143/RConn1 -- Cartesian Joint48/LConn2
  Simulink-PS Converter126/RConn1 -- Cartesian Joint44/LConn4
  Simulink-PS Converter131/RConn1 -- Cartesian Joint42/LConn3
  Simulink-PS Converter133/RConn1 -- Cartesian Joint42/LConn2
  Simulink-PS Converter142/RConn1 -- Cartesian Joint49/LConn4
  Simulink-PS Converter132/RConn1 -- Cartesian Joint42/LConn4
  Simulink-PS Converter140/RConn1 -- Cartesian Joint49/LConn2
  Simulink-PS Converter141/RConn1 -- Cartesian Joint49/LConn3
  Simulink-PS Converter127/RConn1 -- Cartesian Joint44/LConn2
  Simulink-PS Converter145/RConn1 -- Cartesian Joint48/LConn4
  Simulink-PS Converter122/RConn1 -- Cartesian Joint45/LConn3
  Graphic44/RConn1 -- Cartesian Joint42/RConn1
  Graphic42/RConn1 -- Cartesian Joint49/RConn1
  Simulink-PS Converter128/RConn1 -- Cartesian Joint43/LConn3
  Graphic45/RConn1 -- Cartesian Joint43/RConn1
  Simulink-PS Converter139/RConn1 -- Cartesian Joint40/LConn2
  Simulink-PS Converter146/RConn1 -- Cartesian Joint47/LConn2
  Simulink-PS Converter137/RConn1 -- Cartesian Joint40/LConn3
  Simulink-PS Converter123/RConn1 -- Cartesian Joint45/LConn4
  Graphic41/RConn1 -- Cartesian Joint40/RConn1
  Simulink-PS Converter124/RConn1 -- Cartesian Joint45/LConn2
  Simulink-PS Converter134/RConn1 -- Cartesian Joint41/LConn3
  Simulink-PS Converter121/RConn1 -- Cartesian Joint46/LConn4
  Simulink-PS Converter120/RConn1 -- Cartesian Joint46/LConn3
  Graphic48/RConn1 -- Cartesian Joint46/RConn1
  Graphic50/RConn1 -- Cartesian Joint48/RConn1
  Simulink-PS Converter129/RConn1 -- Cartesian Joint43/LConn4
  Simulink-PS Converter136/RConn1 -- Cartesian Joint41/LConn2
  Graphic47/RConn1 -- Cartesian Joint45/RConn1
  Simulink-PS Converter138/RConn1 -- Cartesian Joint40/LConn4
  Graphic46/RConn1 -- Cartesian Joint44/RConn1
  Graphic43/RConn1 -- Cartesian Joint41/RConn1
  Simulink-PS Converter125/RConn1 -- Cartesian Joint44/LConn3
  Simulink-PS Converter135/RConn1 -- Cartesian Joint41/LConn4
  Simulink-PS Converter149/RConn1 -- Cartesian Joint46/LConn2
  Simulink-PS Converter130/RConn1 -- Cartesian Joint43/LConn2
  Simulink-PS Converter148/RConn1 -- Cartesian Joint47/LConn4
  Graphic49/RConn1 -- Cartesian Joint47/RConn1
  Simulink-PS Converter147/RConn1 -- Cartesian Joint47/LConn3
  Simulink-PS Converter144/RConn1 -- Cartesian Joint48/LConn3
  Simulink-PS Converter173/RConn1 -- Cartesian Joint58/LConn2
  Simulink-PS Converter156/RConn1 -- Cartesian Joint54/LConn4
  Simulink-PS Converter161/RConn1 -- Cartesian Joint52/LConn3
  Simulink-PS Converter163/RConn1 -- Cartesian Joint52/LConn2
  Simulink-PS Converter172/RConn1 -- Cartesian Joint59/LConn4
  Simulink-PS Converter162/RConn1 -- Cartesian Joint52/LConn4
  Simulink-PS Converter170/RConn1 -- Cartesian Joint59/LConn2
  Simulink-PS Converter171/RConn1 -- Cartesian Joint59/LConn3
  Simulink-PS Converter157/RConn1 -- Cartesian Joint54/LConn2
  Simulink-PS Converter175/RConn1 -- Cartesian Joint58/LConn4
  Simulink-PS Converter152/RConn1 -- Cartesian Joint55/LConn3
  Graphic54/RConn1 -- Cartesian Joint52/RConn1
  Graphic52/RConn1 -- Cartesian Joint59/RConn1
  Simulink-PS Converter158/RConn1 -- Cartesian Joint53/LConn3
  Graphic55/RConn1 -- Cartesian Joint53/RConn1
  Simulink-PS Converter169/RConn1 -- Cartesian Joint50/LConn2
  Simulink-PS Converter176/RConn1 -- Cartesian Joint57/LConn2
  Simulink-PS Converter167/RConn1 -- Cartesian Joint50/LConn3
  Simulink-PS Converter153/RConn1 -- Cartesian Joint55/LConn4
  Graphic51/RConn1 -- Cartesian Joint50/RConn1
  Simulink-PS Converter154/RConn1 -- Cartesian Joint55/LConn2
  Simulink-PS Converter164/RConn1 -- Cartesian Joint51/LConn3
  Simulink-PS Converter151/RConn1 -- Cartesian Joint56/LConn4
  Simulink-PS Converter150/RConn1 -- Cartesian Joint56/LConn3
  Graphic58/RConn1 -- Cartesian Joint56/RConn1
  Graphic60/RConn1 -- Cartesian Joint58/RConn1
  Simulink-PS Converter159/RConn1 -- Cartesian Joint53/LConn4
  Simulink-PS Converter166/RConn1 -- Cartesian Joint51/LConn2
  Graphic57/RConn1 -- Cartesian Joint55/RConn1
  Simulink-PS Converter168/RConn1 -- Cartesian Joint50/LConn4
  Graphic56/RConn1 -- Cartesian Joint54/RConn1
  Graphic53/RConn1 -- Cartesian Joint51/RConn1
  Simulink-PS Converter155/RConn1 -- Cartesian Joint54/LConn3
  Simulink-PS Converter165/RConn1 -- Cartesian Joint51/LConn4
  Simulink-PS Converter179/RConn1 -- Cartesian Joint56/LConn2
  Simulink-PS Converter160/RConn1 -- Cartesian Joint53/LConn2
  Simulink-PS Converter178/RConn1 -- Cartesian Joint57/LConn4
  Graphic59/RConn1 -- Cartesian Joint57/RConn1
  Simulink-PS Converter177/RConn1 -- Cartesian Joint57/LConn3
  Simulink-PS Converter174/RConn1 -- Cartesian Joint58/LConn3
  Simulink-PS Converter203/RConn1 -- Cartesian Joint68/LConn2
  Simulink-PS Converter186/RConn1 -- Cartesian Joint64/LConn4
  Simulink-PS Converter191/RConn1 -- Cartesian Joint62/LConn3
  Simulink-PS Converter193/RConn1 -- Cartesian Joint62/LConn2
  Simulink-PS Converter202/RConn1 -- Cartesian Joint69/LConn4
  Simulink-PS Converter192/RConn1 -- Cartesian Joint62/LConn4
  Simulink-PS Converter200/RConn1 -- Cartesian Joint69/LConn2
  Simulink-PS Converter201/RConn1 -- Cartesian Joint69/LConn3
  Simulink-PS Converter187/RConn1 -- Cartesian Joint64/LConn2
  Simulink-PS Converter205/RConn1 -- Cartesian Joint68/LConn4
  Simulink-PS Converter182/RConn1 -- Cartesian Joint65/LConn3
  Graphic64/RConn1 -- Cartesian Joint62/RConn1
  Graphic62/RConn1 -- Cartesian Joint69/RConn1
  Simulink-PS Converter188/RConn1 -- Cartesian Joint63/LConn3
  Graphic65/RConn1 -- Cartesian Joint63/RConn1
  Simulink-PS Converter199/RConn1 -- Cartesian Joint60/LConn2
  Simulink-PS Converter206/RConn1 -- Cartesian Joint67/LConn2
  Simulink-PS Converter197/RConn1 -- Cartesian Joint60/LConn3
  Simulink-PS Converter183/RConn1 -- Cartesian Joint65/LConn4
  Graphic61/RConn1 -- Cartesian Joint60/RConn1
  Simulink-PS Converter184/RConn1 -- Cartesian Joint65/LConn2
  Simulink-PS Converter194/RConn1 -- Cartesian Joint61/LConn3
  Simulink-PS Converter181/RConn1 -- Cartesian Joint66/LConn4
  Simulink-PS Converter180/RConn1 -- Cartesian Joint66/LConn3
  Graphic68/RConn1 -- Cartesian Joint66/RConn1
  Graphic70/RConn1 -- Cartesian Joint68/RConn1
  Simulink-PS Converter189/RConn1 -- Cartesian Joint63/LConn4
  Simulink-PS Converter196/RConn1 -- Cartesian Joint61/LConn2
  Graphic67/RConn1 -- Cartesian Joint65/RConn1
  Simulink-PS Converter198/RConn1 -- Cartesian Joint60/LConn4
  Graphic66/RConn1 -- Cartesian Joint64/RConn1
  Graphic63/RConn1 -- Cartesian Joint61/RConn1
  Simulink-PS Converter185/RConn1 -- Cartesian Joint64/LConn3
  Simulink-PS Converter195/RConn1 -- Cartesian Joint61/LConn4
  Simulink-PS Converter209/RConn1 -- Cartesian Joint66/LConn2
  Simulink-PS Converter190/RConn1 -- Cartesian Joint63/LConn2
  Simulink-PS Converter208/RConn1 -- Cartesian Joint67/LConn4
  Graphic69/RConn1 -- Cartesian Joint67/RConn1
  Simulink-PS Converter207/RConn1 -- Cartesian Joint67/LConn3
  Simulink-PS Converter204/RConn1 -- Cartesian Joint68/LConn3
  Simulink-PS Converter233/RConn1 -- Cartesian Joint78/LConn2
  Simulink-PS Converter216/RConn1 -- Cartesian Joint74/LConn4
  Simulink-PS Converter221/RConn1 -- Cartesian Joint72/LConn3
  Simulink-PS Converter223/RConn1 -- Cartesian Joint72/LConn2
  Simulink-PS Converter232/RConn1 -- Cartesian Joint79/LConn4
  Simulink-PS Converter222/RConn1 -- Cartesian Joint72/LConn4
  Simulink-PS Converter230/RConn1 -- Cartesian Joint79/LConn2
  Simulink-PS Converter231/RConn1 -- Cartesian Joint79/LConn3
  Simulink-PS Converter217/RConn1 -- Cartesian Joint74/LConn2
  Simulink-PS Converter235/RConn1 -- Cartesian Joint78/LConn4
  Simulink-PS Converter212/RConn1 -- Cartesian Joint75/LConn3
  Graphic74/RConn1 -- Cartesian Joint72/RConn1
  Graphic72/RConn1 -- Cartesian Joint79/RConn1
  Simulink-PS Converter218/RConn1 -- Cartesian Joint73/LConn3
  Graphic75/RConn1 -- Cartesian Joint73/RConn1
  Simulink-PS Converter229/RConn1 -- Cartesian Joint70/LConn2
  Simulink-PS Converter236/RConn1 -- Cartesian Joint77/LConn2
  Simulink-PS Converter227/RConn1 -- Cartesian Joint70/LConn3
  Simulink-PS Converter213/RConn1 -- Cartesian Joint75/LConn4
  Graphic71/RConn1 -- Cartesian Joint70/RConn1
  Simulink-PS Converter214/RConn1 -- Cartesian Joint75/LConn2
  Simulink-PS Converter224/RConn1 -- Cartesian Joint71/LConn3
  Simulink-PS Converter211/RConn1 -- Cartesian Joint76/LConn4
  Simulink-PS Converter210/RConn1 -- Cartesian Joint76/LConn3
  Graphic78/RConn1 -- Cartesian Joint76/RConn1
  Graphic80/RConn1 -- Cartesian Joint78/RConn1
  Simulink-PS Converter219/RConn1 -- Cartesian Joint73/LConn4
  Simulink-PS Converter226/RConn1 -- Cartesian Joint71/LConn2
  Graphic77/RConn1 -- Cartesian Joint75/RConn1
  Simulink-PS Converter228/RConn1 -- Cartesian Joint70/LConn4
  Graphic76/RConn1 -- Cartesian Joint74/RConn1
  Graphic73/RConn1 -- Cartesian Joint71/RConn1
  Simulink-PS Converter215/RConn1 -- Cartesian Joint74/LConn3
  Simulink-PS Converter225/RConn1 -- Cartesian Joint71/LConn4
  Simulink-PS Converter239/RConn1 -- Cartesian Joint76/LConn2
  Simulink-PS Converter220/RConn1 -- Cartesian Joint73/LConn2
  Simulink-PS Converter238/RConn1 -- Cartesian Joint77/LConn4
  Graphic79/RConn1 -- Cartesian Joint77/RConn1
  Simulink-PS Converter237/RConn1 -- Cartesian Joint77/LConn3
  Simulink-PS Converter234/RConn1 -- Cartesian Joint78/LConn3
  Simulink-PS Converter263/RConn1 -- Cartesian Joint88/LConn2
  Simulink-PS Converter246/RConn1 -- Cartesian Joint84/LConn4
  Simulink-PS Converter251/RConn1 -- Cartesian Joint82/LConn3
  Simulink-PS Converter253/RConn1 -- Cartesian Joint82/LConn2
  Simulink-PS Converter262/RConn1 -- Cartesian Joint89/LConn4
  Simulink-PS Converter252/RConn1 -- Cartesian Joint82/LConn4
  Simulink-PS Converter260/RConn1 -- Cartesian Joint89/LConn2
  Simulink-PS Converter261/RConn1 -- Cartesian Joint89/LConn3
  Simulink-PS Converter247/RConn1 -- Cartesian Joint84/LConn2
  Simulink-PS Converter265/RConn1 -- Cartesian Joint88/LConn4
  Simulink-PS Converter242/RConn1 -- Cartesian Joint85/LConn3
  Graphic84/RConn1 -- Cartesian Joint82/RConn1
  Graphic82/RConn1 -- Cartesian Joint89/RConn1
  Simulink-PS Converter248/RConn1 -- Cartesian Joint83/LConn3
  Graphic85/RConn1 -- Cartesian Joint83/RConn1
  Simulink-PS Converter259/RConn1 -- Cartesian Joint80/LConn2
  Simulink-PS Converter266/RConn1 -- Cartesian Joint87/LConn2
  Simulink-PS Converter257/RConn1 -- Cartesian Joint80/LConn3
  Simulink-PS Converter243/RConn1 -- Cartesian Joint85/LConn4
  Graphic81/RConn1 -- Cartesian Joint80/RConn1
  Simulink-PS Converter244/RConn1 -- Cartesian Joint85/LConn2
  Simulink-PS Converter254/RConn1 -- Cartesian Joint81/LConn3
  Simulink-PS Converter241/RConn1 -- Cartesian Joint86/LConn4
  Simulink-PS Converter240/RConn1 -- Cartesian Joint86/LConn3
  Graphic88/RConn1 -- Cartesian Joint86/RConn1
  Graphic90/RConn1 -- Cartesian Joint88/RConn1
  Simulink-PS Converter249/RConn1 -- Cartesian Joint83/LConn4
  Simulink-PS Converter256/RConn1 -- Cartesian Joint81/LConn2
  Graphic87/RConn1 -- Cartesian Joint85/RConn1
  Simulink-PS Converter258/RConn1 -- Cartesian Joint80/LConn4
  Graphic86/RConn1 -- Cartesian Joint84/RConn1
  Graphic83/RConn1 -- Cartesian Joint81/RConn1
  Simulink-PS Converter245/RConn1 -- Cartesian Joint84/LConn3
  Simulink-PS Converter255/RConn1 -- Cartesian Joint81/LConn4
  Simulink-PS Converter269/RConn1 -- Cartesian Joint86/LConn2
  Simulink-PS Converter250/RConn1 -- Cartesian Joint83/LConn2
  Simulink-PS Converter268/RConn1 -- Cartesian Joint87/LConn4
  Graphic89/RConn1 -- Cartesian Joint87/RConn1
  Simulink-PS Converter267/RConn1 -- Cartesian Joint87/LConn3
  Simulink-PS Converter264/RConn1 -- Cartesian Joint88/LConn3
  Simulink-PS Converter293/RConn1 -- Cartesian Joint98/LConn2
  Simulink-PS Converter276/RConn1 -- Cartesian Joint94/LConn4
  Simulink-PS Converter281/RConn1 -- Cartesian Joint92/LConn3
  Simulink-PS Converter283/RConn1 -- Cartesian Joint92/LConn2
  Simulink-PS Converter292/RConn1 -- Cartesian Joint99/LConn4
  Simulink-PS Converter282/RConn1 -- Cartesian Joint92/LConn4
  Simulink-PS Converter290/RConn1 -- Cartesian Joint99/LConn2
  Simulink-PS Converter291/RConn1 -- Cartesian Joint99/LConn3
  Simulink-PS Converter277/RConn1 -- Cartesian Joint94/LConn2
  Simulink-PS Converter295/RConn1 -- Cartesian Joint98/LConn4
  Simulink-PS Converter272/RConn1 -- Cartesian Joint95/LConn3
  Graphic94/RConn1 -- Cartesian Joint92/RConn1
  Graphic92/RConn1 -- Cartesian Joint99/RConn1
  Simulink-PS Converter278/RConn1 -- Cartesian Joint93/LConn3
  Graphic95/RConn1 -- Cartesian Joint93/RConn1
  Simulink-PS Converter289/RConn1 -- Cartesian Joint90/LConn2
  Simulink-PS Converter296/RConn1 -- Cartesian Joint97/LConn2
  Simulink-PS Converter287/RConn1 -- Cartesian Joint90/LConn3
  Simulink-PS Converter273/RConn1 -- Cartesian Joint95/LConn4
  Graphic91/RConn1 -- Cartesian Joint90/RConn1
  Simulink-PS Converter274/RConn1 -- Cartesian Joint95/LConn2
  Simulink-PS Converter284/RConn1 -- Cartesian Joint91/LConn3
  Simulink-PS Converter271/RConn1 -- Cartesian Joint96/LConn4
  Simulink-PS Converter270/RConn1 -- Cartesian Joint96/LConn3
  Graphic98/RConn1 -- Cartesian Joint96/RConn1
  Graphic100/RConn1 -- Cartesian Joint98/RConn1
  Simulink-PS Converter279/RConn1 -- Cartesian Joint93/LConn4
  Simulink-PS Converter286/RConn1 -- Cartesian Joint91/LConn2
  Graphic97/RConn1 -- Cartesian Joint95/RConn1
  Simulink-PS Converter288/RConn1 -- Cartesian Joint90/LConn4
  Graphic96/RConn1 -- Cartesian Joint94/RConn1
  Graphic93/RConn1 -- Cartesian Joint91/RConn1
  Simulink-PS Converter275/RConn1 -- Cartesian Joint94/LConn3
  Simulink-PS Converter285/RConn1 -- Cartesian Joint91/LConn4
  Simulink-PS Converter299/RConn1 -- Cartesian Joint96/LConn2
  Simulink-PS Converter280/RConn1 -- Cartesian Joint93/LConn2
  Simulink-PS Converter298/RConn1 -- Cartesian Joint97/LConn4
  Graphic99/RConn1 -- Cartesian Joint97/RConn1
  Simulink-PS Converter297/RConn1 -- Cartesian Joint97/LConn3
  Simulink-PS Converter294/RConn1 -- Cartesian Joint98/LConn3
